simulink model "prj5"  (R2021a)
settings: Solver=VariableStepAuto  StartTime=0.0  StopTime=300  RelTol=1e-3
undefined symbols (not defined in the file or in its folder): AXI4, Lite
libraries: hdlBasic x33, prj5pelib x6, xbsIndex_r4 x1
settings Model: Creator=asc8  LastModifiedBy=asc8

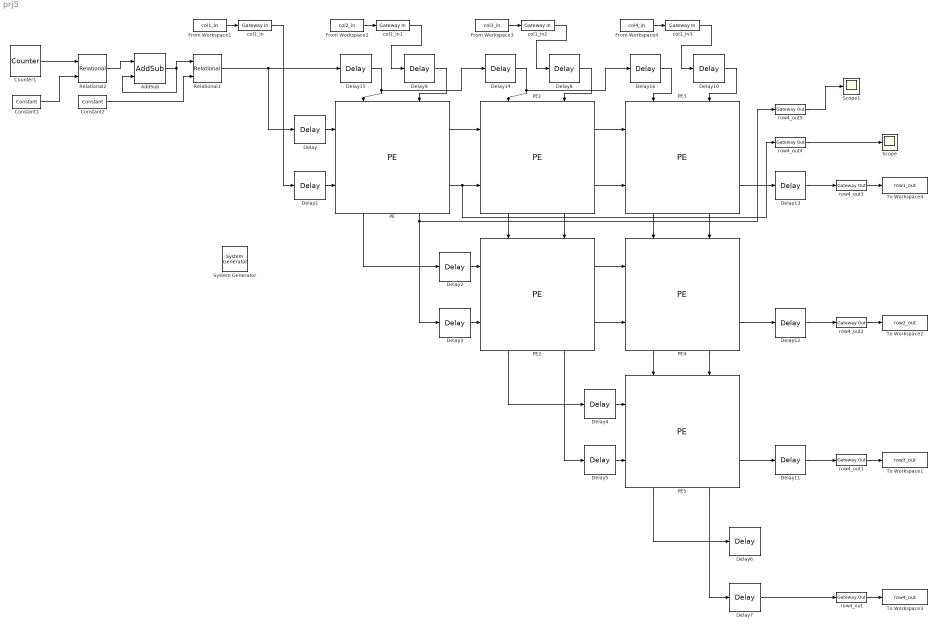
== system prj5 ==
  " System Generator" : xbsIndex_r4/ System Generator  Tag=genX  xilinxfamily=kintex7  part=xc7k325t  speed=-3  package=fbg676  synthesis_tool=Vivado  clock_wrapper=Clock Enables  directory=./netlist  proj_type=Vivado  Synth_file=Vivado Synthesis Defaults  Impl_file=Vivado Implementation Defaults  testbench=off  simulink_period=1  sysclk_period=10  dcm_input_clock_period=10  incr_netlist=off  trim_vbits=Everywhere in SubSystem  dbl_ovrd=According to Block Masks  core_generation=According to Block Masks  run_coregen=off  deprecated_control=off  eval_field=0  block_type=sysgen
  AddSub : hdlBasic/AddSub  mode=Addition  use_carryin=off  use_carryout=off  en=off  latency=1  precision=User Defined  arith_type=Unsigned  n_bits=3  bin_pt=0  quantization=Truncate  overflow=Wrap  use_behavioral_HDL=off  hw_selection=Fabric  pipelined=off  XmcBlockStatus=1  maskContainerNames=tabcontainer1  block_type=addsub  block_config=sysgen:Addsub_config
  Constant1 : hdlBasic/Constant  const=19  gui_display_data_type=Fixed-point  arith_type=Unsigned  n_bits=8  bin_pt=0  preci_type=Single  exp_width=8  frac_width=24  explicit_period=off  period=1  XmcBlockStatus=1  maskContainerNames=tabcontainer1  block_type=constant  block_config=sysgen:Constant_config
  Constant2 : hdlBasic/Constant  const=0  gui_display_data_type=Fixed-point  arith_type=Unsigned  n_bits=3  bin_pt=0  preci_type=Single  exp_width=8  frac_width=24  explicit_period=off  period=1  XmcBlockStatus=1  maskContainerNames=tabcontainer1  block_type=constant  block_config=sysgen:Constant_config
  Counter1 : hdlBasic/Counter  cnt_type=Count limited  cnt_to=19  operation=Up  start_count=0  cnt_by_val=1  arith_type=Unsigned  n_bits=8  bin_pt=0  load_pin=off  rst=off  en=off  explicit_period=Explicit  period=1  use_behavioral_HDL=off  implementation=Fabric  XmcBlockStatus=1  maskContainerNames=group1  block_type=counter  block_config=sysgen:Counter_config
  Delay{,1..7,9,11} (10 alike) : hdlBasic/Delay  rst=off  en=off  latency=20  reg_retiming=off  XmcBlockStatus=1  maskContainerNames=group1  block_type=delay  block_config=sysgen:Delay_config
  Delay10 : hdlBasic/Delay  rst=off  en=off  latency=60  reg_retiming=off  XmcBlockStatus=1  maskContainerNames=group1  block_type=delay  block_config=sysgen:Delay_config
  Delay{8,12,14..16} (5 alike) : hdlBasic/Delay  rst=off  en=off  latency=40  reg_retiming=off  XmcBlockStatus=1  maskContainerNames=group1  block_type=delay  block_config=sysgen:Delay_config
  Delay13 : hdlBasic/Delay  rst=off  en=off  latency=60  reg_retiming=off  XmcBlockStatus=1  maskContainerNames=group1  block_type=delay  block_config=sysgen:Delay_config
  From Workspace1 : FromWorkspace  VariableName=col1_in
  From Workspace2 : FromWorkspace  VariableName=col2_in
  From Workspace3 : FromWorkspace  VariableName=col3_in
  From Workspace4 : FromWorkspace  VariableName=col4_in
  PE{,1..5} (6 alike) : prj5pelib/PE  SystemSampleTime=-1  VariantActivationTime=update diagram  Latency=0  AutoFrameSizeCalculation=off
      settings: SourceProductName=Aedan's Project 5 PE Library  PortSchema="{\"entries\":[{\"content\":{\"sides\":[{\"content\":{\"connectorIds\":[\"In1\",\"In2\"]},\"type\":\"ConnectorPlacement.EquallySpacedRectSide\",\"uuid\":\"f7e55443-70fb-4ed5-ab4f-147f7311106a\"},{\"content\":{\"connectorIds\":[\"Out1\",\"Out2\"],\"side\":\"RIGHT\"},\"type\":\"ConnectorPlacement.EquallySpacedRectSide\",\"uuid\":\"6de0769a-4a22-4abb-b630-26d0c175204f\"},{\"content\":{\"connectorIds\":[\"In3\",\"In4\"],\"side\":\"TOP\"},\"type\":\"ConnectorPlacement.EquallySpacedRectSide\",\"uuid\":\"a041cc58-78e8-4444-b053-dd6f2c27badd\"},{\"content\":{\"connectorIds\":[\"Out3\",\"Out4\"],\"side\":\"BOTTOM\"},\"type\":\"ConnectorPlacement.EquallySpacedRectSide\",\"uuid\":\"085ff6f5-8624-4aab-b622-9beedcd77ebd\"}]},\"type\":\"ConnectorPlacement.EquallySpacedConnector\",\"uuid\":\"928950cd-8b9e-4ebf-b8fd-b98c3e494fdc\"}],\"packageUris\":[\"http://schema.mathworks.com/mf0/Connector/R2020b\"],\"version\":\"1.0\"}"
  Relational1 : hdlBasic/Relational  mode=a=b  op_type=Bool  en=off  latency=0  XmcBlockStatus=1  maskContainerNames=tabcontainer1  block_type=relational  block_config=sysgen:Relational_config
  Relational2 : hdlBasic/Relational  mode=a=b  op_type=Unsigned Fix  en=off  latency=0  XmcBlockStatus=1  maskContainerNames=tabcontainer1  block_type=relational  block_config=sysgen:Relational_config
  Scope : Scope
  Scope1 : Scope
  To Workspace1 : ToWorkspace  VariableName=row3_out  SaveFormat=Timeseries  SampleTime=-1
  To Workspace2 : ToWorkspace  VariableName=row2_out  SaveFormat=Timeseries  SampleTime=-1
  To Workspace3 : ToWorkspace  VariableName=row4_out  SaveFormat=Timeseries  SampleTime=-1
  To Workspace4 : ToWorkspace  VariableName=row1_out  SaveFormat=Timeseries  SampleTime=-1
  col1_in{,1..3} (4 alike) : hdlBasic/Gateway In  gui_display_data_type=Fixed-point  arith_type=Signed (2's comp)  n_bits=16  bin_pt=12  preci_type=Single  exp_width=8  frac_width=24  rows=1  columns=1  quantization="Round  (unbiased: +/- Inf)"  overflow=Saturate  period=1  UseAsADC=off  ADCChannel='1'  interface=AXI4-Lite  automatic_assignment=on  address_offset=hex2dec('00')  intf_name=''  intf_description=''  default_value=0  timing_constraint=None  locs_specified=off  LOCs={}  io_standard={}  inherit_from_input=off  hdl_port=on  XmcBlockStatus=1  maskContainerNames=group4  block_type=gatewayin  block_config=sysgen:gateway_in_config  block_width_w=590  block_height_w=620  block_width=640  block_height=850
  row4_out{,1..5} (6 alike) : hdlBasic/Gateway Out  inherit_from_input=off  hdl_port=on  rows=1  columns=1  UseAsDAC=off  DACChannel='1'  interface=AXI4-Lite  automatic_assignment=on  address_offset=hex2dec('00')  intf_name=''  intf_description=''  timing_constraint=None  locs_specified=off  LOCs={}  io_standard={}  XmcBlockStatus=1  maskContainerNames=group4  block_type=gatewayout  block_config=sysgen:gateway_out_config  block_width_w=590  block_height_w=620  block_width=620  block_height=750
  wires:
  PE/1 -> PE1/1
  PE/2 -> row4_out4/1, PE1/2
  PE1/3 -> PE2/3
  PE1/4 -> PE2/4
  PE1/2 -> PE3/2
  PE1/1 -> PE3/1
  PE2/1 -> PE4/1
  PE2/2 -> PE4/2
  PE3/3 -> PE4/3
  PE3/4 -> PE4/4
  PE4/3 -> PE5/3
  PE4/4 -> PE5/4
  Delay/1 -> PE/1
  Delay1/1 -> PE/2
  Delay2/1 -> PE2/1
  Delay3/1 -> PE2/2
  PE/3 -> Delay2/1
  PE/4 -> row4_out5/1, Delay3/1
  Delay4/1 -> PE5/1
  Delay5/1 -> PE5/2
  PE2/3 -> Delay4/1
  PE2/4 -> Delay5/1
  PE5/3 -> Delay6/1
  PE5/4 -> Delay7/1
  Delay8/1 -> PE1/4
  Delay9/1 -> PE/4
  Delay10/1 -> PE3/4
  From Workspace1/1 -> col1_in/1
  From Workspace2/1 -> col1_in1/1
  From Workspace3/1 -> col1_in2/1
  col1_in1/1 -> Delay9/1
  col1_in2/1 -> Delay8/1
  From Workspace4/1 -> col1_in3/1
  col1_in3/1 -> Delay10/1
  row4_out/1 -> To Workspace3/1
  Delay7/1 -> row4_out/1
  row4_out1/1 -> To Workspace1/1
  Delay11/1 -> row4_out1/1
  PE5/2 -> Delay11/1
  Delay12/1 -> row4_out2/1
  row4_out2/1 -> To Workspace2/1
  PE4/2 -> Delay12/1
  Delay13/1 -> row4_out3/1
  PE3/2 -> Delay13/1
  Delay14/1 -> PE1/3, Delay16/1
  Delay15/1 -> PE/3, Delay14/1
  Delay16/1 -> PE3/3
  col1_in/1 -> Delay1/1
  Relational1/1 -> Delay/1, Delay15/1
  Relational2/1 -> AddSub/1
  Counter1/1 -> Relational2/1
  AddSub/1 -> Relational1/1, AddSub/2
  Constant1/1 -> Relational2/2
  Constant2/1 -> Relational1/2
  row4_out3/1 -> To Workspace4/1
  row4_out4/1 -> Scope/1
  row4_out5/1 -> Scope1/1
